simulink model "zmp_com"  (R2023b)
settings: Solver=ode4  StartTime=0.0  StopTime=t_stop  RelTol=1e-3
settings Model: Creator=Vedang  LastModifiedBy=Vedang

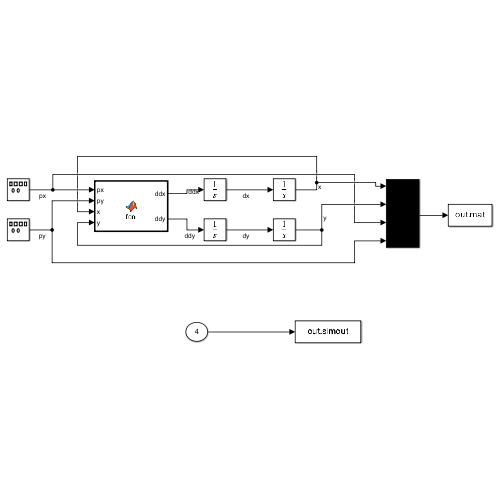
[thumbnail: Simulink's stored preview of the top-level diagram]
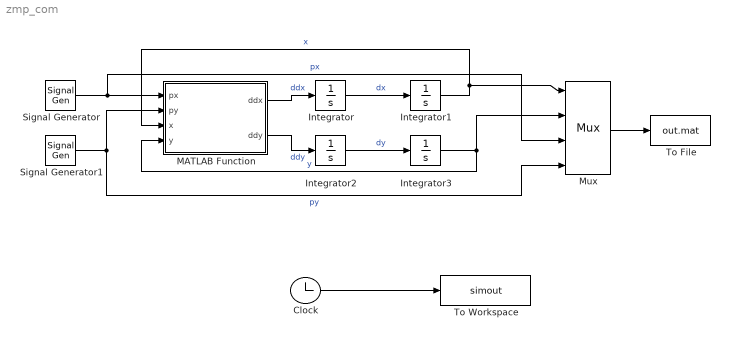
== system zmp_com ==
  Clock : Clock
  Integrator{,1..3} (4 alike) : Integrator
  MATLAB Function : MATLAB Function  TreatAsAtomicUnit=on
  Mux : Mux
  Signal Generator : SignalGenerator  WaveForm=square  Amplitude=0.3  Frequency=0.33  Units=rad/sec
  Signal Generator1 : SignalGenerator  WaveForm=square  Amplitude=0.3  Frequency=0.33  Units=rad/sec
  To File : ToFile  Filename=out.mat
  To Workspace : ToWorkspace  VariableName=simout  SaveFormat=Timeseries  SampleTime=-1
  wires:
  Integrator/1 -> Integrator1/1  "dx"
  Integrator2/1 -> Integrator3/1  "dy"
  Integrator1/1 -> MATLAB Function/3(x), Mux/1  "x"
  MATLAB Function/1(ddx) -> Integrator/1  "ddx"
  MATLAB Function/2(ddy) -> Integrator2/1  "ddy"
  Integrator3/1 -> MATLAB Function/4(y), Mux/2  "y"
  Mux/1 -> To File/1
  Signal Generator/1 -> Mux/3, MATLAB Function/1(px)  "px"
  Signal Generator1/1 -> Mux/4, MATLAB Function/2(py)  "py"
  Clock/1 -> To Workspace/1

== matlab function zmp_com/MATLAB Function ==
  data: px input; ddx output; py input; ddy output; x input; y input
function [ddx,ddy] = fcn(px,py,x,y)
g=9.8;
zc= 0.154;
ddx = (g/zc)*(x-px);
ddy = (g/zc)*(y-py);
